simulink subsystem "Gyroscope"  (R2025b)
settings: Solver=VariableStepAuto  StartTime=0.0  StopTime=10.0  RelTol=1e-3
settings Model: Creator=yvijay  LastModifiedBy=YuktiVijay

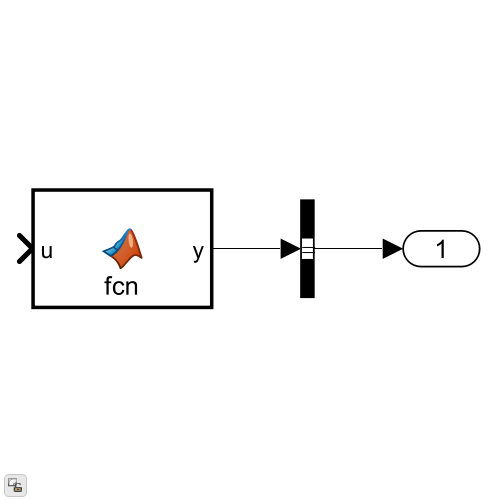
[thumbnail: Simulink's stored preview of the top-level diagram]
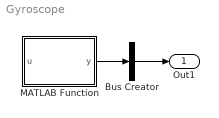
== system Gyroscope ==
  Bus Creator : BusCreator  Inputs=1
  MATLAB Function : MATLAB Function  TreatAsAtomicUnit=on
  Out1 : Outport
  wires:
  MATLAB Function/1(y) -> Bus Creator/1
  Bus Creator/1 -> Out1/1

== matlab function Gyroscope/MATLAB Function ==
  data: u input; y output
function y = fcn(u)

y = u;
